simulink model "orbitSIM"  (R2015a)
settings: Solver=ode113  StartTime=0.0  StopTime=numDaysSim*24*3600  MaxStep=1*60  RelTol=1e-6  AbsTol=1e-9
values from neighbouring files (symbols this model uses):
  a0 = 6776    [PS1.m]    (also in PS4.m; PS5.m; PS7.m)
  B = Cd*A/M    (= 0)    [PS1.m]    (also in PS4.m; fullStateController.m = eye(7); getQuat_dot.m = [0 w(3) -w(2) w(1); -w(3) 0 w(1) w(2); w(2) -w(1) 0 w(3);   ; linearEuler.m = (dt * B_))
  e0 = 0.0004758    [PS1.m]    (also in PS4.m; PS5.m; PS7.m)
  H = 10    [PS1.m]    (also in PS4.m; getRho.m)
  h0 = Re    (= 6371)    [PS1.m]    (also in PS4.m; getRho.m = 6378.137)
  incl0 = 51.6397    [PS1.m]    (also in PS4.m = 0; PS5.m = 0; PS7.m = 0)
  J2 = 0    [PS1.m]    (also in PS4.m; PS5.m; PS7.m)
  mu = 3.986e14 / 1000^3    (= 398600)    [PS1.m]    (also in PS4.m; PS5.m; PS7.m)
  nu0 = 0    [PS1.m]    (also in PS4.m; PS5.m; PS7.m)
  OMEGA0 = 106.0758    [PS1.m]    (also in PS4.m = 0; PS5.m = 0; PS7.m = 0)
  omega0 = 233.6745    [PS1.m]    (also in PS4.m = 0; PS5.m = 0; PS7.m = 0)
  Re = 6371    [PS1.m]    (also in PS4.m; PS5.m; PS7.m)
  rho0 = 1.225*1000^3    (= 1225000000)    [PS1.m]    (also in PS4.m; PS5.m; PS7.m; getRho.m)
  wEarth0 = [0 0 7.292116e-5]'    [PS1.m]    (also in PS4.m)
settings Model: Creator=Toby  LastModifiedBy=Toby
settings DataIOCC: SaveTime=off

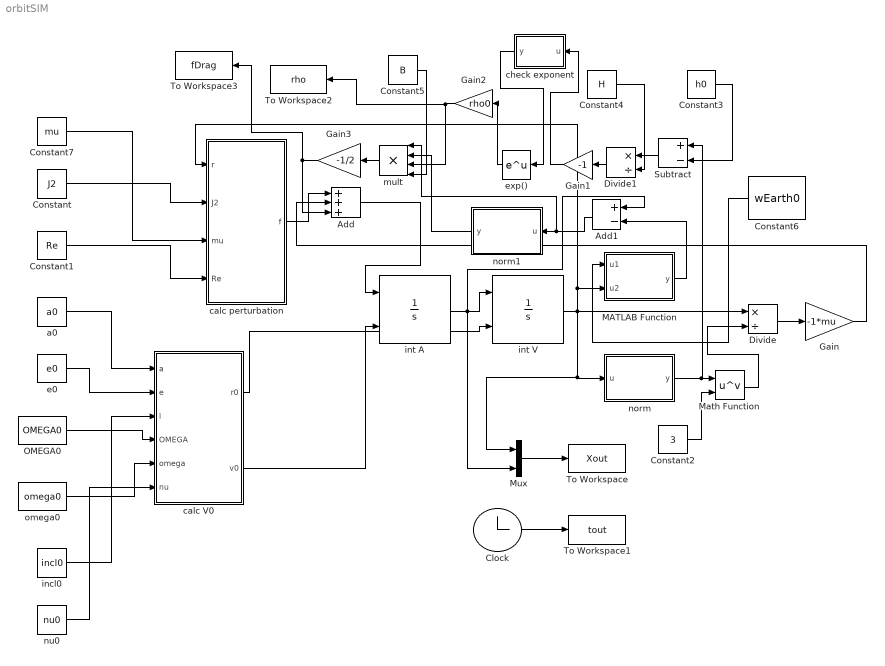
== system orbitSIM ==
  Add : Sum  Inputs=+++
  Add1 : Sum  Inputs=+-
  Clock : Clock
  Constant : Constant  Value=J2
  Constant1 : Constant  Value=Re
  Constant2 : Constant  Value=3
  Constant3 : Constant  Value=h0
  Constant4 : Constant  Value=H
  Constant5 : Constant  Value=B
  Constant6 : Constant  Value=wEarth0
  Constant7 : Constant  Value=mu
  Divide : Product  Inputs=*/
  Divide1 : Product  Inputs=*/
  Gain : Gain  Gain=-1*mu
  Gain1 : Gain  Gain=-1
  Gain2 : Gain  Gain=rho0
  Gain3 : Gain  Gain=-1/2
  MATLAB Function : MATLAB Function  TreatAsAtomicUnit=on
  Math Function : Math  Operator=pow  SaturateOnIntegerOverflow=on
  Mux : Mux  Inputs=2
  OMEGA0 : Constant  Value=OMEGA0
  Subtract : Sum  Inputs=+-
  To Workspace : ToWorkspace  VariableName=Xout  SampleTime=-1
  To Workspace1 : ToWorkspace  VariableName=tout  SampleTime=-1
  To Workspace2 : ToWorkspace  VariableName=rho  SampleTime=-1
  To Workspace3 : ToWorkspace  VariableName=fDrag  SampleTime=-1
  a0 : Constant  Value=a0
  calc V0 : MATLAB Function  TreatAsAtomicUnit=on
  calc perturbation : MATLAB Function  TreatAsAtomicUnit=on
  check exponent : MATLAB Function  TreatAsAtomicUnit=on
  e0 : Constant  Value=e0
  exp() : Math  SaturateOnIntegerOverflow=on
  incl0 : Constant  Value=incl0
  int A : Integrator  InitialConditionSource=external
  int V : Integrator  InitialConditionSource=external
  mult : Product  Inputs=****
  norm : MATLAB Function  TreatAsAtomicUnit=on
  norm1 : MATLAB Function  TreatAsAtomicUnit=on
  nu0 : Constant  Value=nu0
  omega0 : Constant  Value=omega0
  wires:
  a0/1 -> calc V0/1(a)
  e0/1 -> calc V0/2(e)
  incl0/1 -> calc V0/3(i)
  OMEGA0/1 -> calc V0/4(OMEGA)
  omega0/1 -> calc V0/5(omega)
  nu0/1 -> calc V0/6(nu)
  calc V0/1(r0) -> int V/2
  calc perturbation/1(f) -> Add/1
  Add/1 -> int A/1
  calc V0/2(v0) -> int A/2
  int A/1 -> Add1/1, Mux/2, int V/1
  int V/1 -> calc perturbation/1(r), MATLAB Function/2(u2), norm/1(u), Mux/1, Divide/1
  Mux/1 -> To Workspace/1
  norm/1(y) -> Subtract/1, Math Function/1
  Constant2/1 -> Math Function/2
  Math Function/1 -> Divide/2
  Divide/1 -> Gain/1
  Gain/1 -> Add/2
  Constant7/1 -> calc perturbation/3(mu)
  Constant/1 -> calc perturbation/2(J2)
  Constant1/1 -> calc perturbation/4(Re)
  Clock/1 -> To Workspace1/1
  Constant3/1 -> Subtract/2
  Subtract/1 -> Divide1/1
  Constant4/1 -> Divide1/2
  Divide1/1 -> Gain1/1
  Gain1/1 -> check exponent/1(u)
  exp()/1 -> Gain2/1
  Gain2/1 -> To Workspace2/1, mult/3
  mult/1 -> Gain3/1
  Gain3/1 -> To Workspace3/1, Add/3
  Constant5/1 -> mult/4
  MATLAB Function/1(y) -> Add1/2
  Add1/1 -> mult/1, norm1/1(u)
  norm1/1(y) -> mult/2
  Constant6/1 -> MATLAB Function/1(u1)
  check exponent/1(y) -> exp()/1

== matlab function orbitSIM/norm ==
  data: u input; y output
function y = fcn(u)
%#codegen

y = norm(u);

== matlab function orbitSIM/calc perturbation ==
  data: r input; f output; J2 input; mu input; Re input
function f = fcn(r, J2, mu, Re)
% NOTE! EVERYTHING IN DEGREES
% 
% fR = -3*mu*J2*Re^2/(2*r^4)*(1-3*sind(incl)^2*sind(u)^2);
% fT = -3*mu*J2*Re^2/(2*r^4)*(sind(incl)^2*sind(u)*cosd(u));
% fN = -3*mu*J2*Re^2/(2*r^4)*(sind(incl)*cosd(incl)*sind(u));
rMag = norm(r);
rDir = r ./ norm(r);
f = -mu*J2*Re^2/2*( [0, 0, 6*r(3)/rMag^5]' + ...
      (3/rMag^4 - 15*(r(3)^2/rMag^6)).*rDir);

end

== matlab function orbitSIM/calc V0 ==
  data: a input; r0 output; e input; i input; OMEGA input; omega input; nu input; v0 output
function [r0, v0] = fcn(a, e, i, OMEGA, omega, nu)
%#codegen
[r0, v0] = OE2XV(a, e, i, OMEGA, omega, nu);
end

== matlab function orbitSIM/norm1 ==
  data: u input; y output
function y = fcn(u)
%#codegen

y = norm(u);

== matlab function orbitSIM/MATLAB Function ==
  data: u1 input; y output; u2 input
function y = fcn(u1,u2)
%#codegen

y = cross(u1,u2);

== matlab function orbitSIM/check exponent ==
  data: u input; y output
function y = fcn(u)
%#codegen
if u>0
  y = 0;
else
  y = u;
end
